simulink model "Final_project_TEMPLATE"  (R2015b)
settings: Solver=FixedStepDiscrete  StartTime=0.0  StopTime=10.0  RelTol=1e-3
InitFcn:
  | parameters
values from neighbouring files (symbols this model uses):
  Ak = 100    [parameters.m]
  b = 100    [parameters.m]
  dc_sathigh = .76    (= 0.76)    [parameters.m]
  dc_satlow = .24    (= 0.24)    [parameters.m]
  dT = 0.01    [parameters.m]
  H = 20    [parameters.m]
  L1 = 1.6    [parameters.m]
  L2 = 0.8    [parameters.m]
  m = 2000    [parameters.m]
  n_desired = 0    [parameters.m]
  pot_gain = 1    [parameters.m]
  pot_offset = 512    [parameters.m]
  R = 1/5    (= 0.2)    [parameters.m]
  S_Kd1 = .045    (= 0.045)    [parameters.m]
  S_Kd2 = 80    [parameters.m]
  S_Ki2 = 0.0001    [parameters.m]
  S_Kp1 = 0.45    [parameters.m]
  S_Kp2 = 600    [parameters.m]
  t2d = 2*pi/4000    (= 0.00157079632679)    [parameters.m]
  V_Ki = 50    [parameters.m]
  V_Kp = 5000    [parameters.m]
undefined symbols (not defined in the file or in its folder): A10, A13, A14, AN0, AN12, B, B13, B4, B6, C6, D, D11, D4, DiscIntNeverNeededParam, F15, F3, F4, G4, H4, L3, M14, N15, PA10, PA11, PA12, PA13, PA14, PA5, PA6, PA7, PA8, PA9, PB10, PB7, PC11, PC12, PC13, PC6, PD11, R10, R16, R5, R8
libraries: Conv_Lib x54, rappid_564xl_ec_toolbox x37, Veh_Sim x9, simulink x2, U_of_M_5643_blockset x1
(part 1 of 2)
settings Model: Creator=cculkin  LastModifiedBy=yiyupan
settings DataIOCC: ExternalInput=off  InitialState=off  SaveOutput=off  SignalLogging=off  SaveTime=off
settings OptimizationCC: DefaultParameterBehavior=Inlined  DataBitsets=on  OptimizeModelRefInitCode=on  LifeSpan=1
settings DebuggingCC: InheritedTsInSrcMsg=none  SingleTaskRateTransMsg=error  UnconnectedInputMsg=error  UnconnectedOutputMsg=error  UnconnectedLineMsg=error  UnknownTsInhSupMsg=error
settings HardwareCC: ProdBitPerPointer=32  ProdLargestAtomicInteger=Long  ProdLargestAtomicFloat=Double  ProdEndianess=BigEndian  ProdWordSize=32  ProdHWDeviceType=Freescale->32-bit PowerPC
settings RTWCC: SystemTargetFile=rappid564xl.tlc  MakeCommand=rappid_564xl_make_rtw  TemplateMakefile=rappid_564xl_default_tmf  PostCodeGenCommand=rappid_analyzegencode(buildInfo)  Description=RAppID Toolbox MPC564xL Code Generation Target (rappid)  GenerateReport=on  IncludeHyperlinkInReport=on  LaunchReport=on
settings CodeAppCC: IgnoreCustomStorageClasses=off
settings STFCustomTargetCC: ModelReferenceCompliant=off  ConcurrentExecutionCompliant=off  GeneratePreprocessorConditionals=Use local settings  CombineOutputUpdateFcns=on  ERTCustomFileBanners=on  SupportContinuousTime=off  SupportNonInlinedSFcns=off  MATLABClassNameForMDSCustomization=Simulink.SoftwareTarget.ERTCustomization  CPPClassGenCompliant=off  GRTInterface=off  SystemTargetFile=rappid564xl.tlc
settings ERTTargetCC: ModelReferenceCompliant=off  ParMdlRefBuildCompliant=off  CompOptLevelCompliant=off  ConcurrentExecutionCompliant=off  ERTFirstTimeCompliant=off  ModelStepFunctionPrototypeControlCompliant=off  CPPClassGenCompliant=off  UseToolchainInfoCompliant=off  InlinedParameterPlacement=NonHierarchical  ERTCustomFileTemplate=example_file_process.tlc

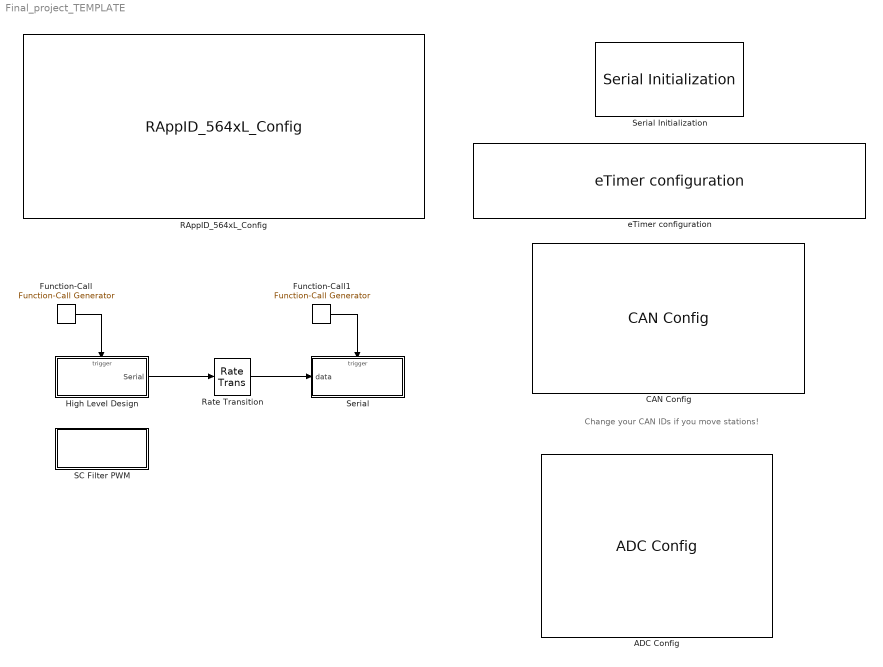
== system Final_project_TEMPLATE ==
  note: Change your CAN IDs if you move stations!
  ADC Config : rappid_564xl_ec_toolbox/MPC564xL/Motor Control Blocks/ADC Config  adc_unit=0  adc_ctu=off  adc_owr=on  adc_wls=Left  adc_clk=on  adc_ack=on  adc_ctr0_inp=off  adc_ctr0_shft=10 - Avin = 0  adc_ctr0_cmp=01  adc_ctr0_samp=3  adc_ctr1_inp=off  adc_ctr1_cmp=01  adc_ctr1_samp=1  adc_ctr1_tsens=PTAT  adc_pscr_preval=V0  adc_pscr_preconv=off
  CAN Config : rappid_564xl_ec_toolbox/MPC564xL/Communication Blocks/CAN Config  Priority=1  can_unit=A  can_unit_v2=0  can_idam=A - One full ID (standard or extended) per filter element.  can_srx_dis=1 - Self reception disabled  can_presdiv=4  can_rjw=3  can_pseg1=5  can_pseg2=5  can_clk_src=0 - The CAN engine clock source is the oscillator clock  can_lpb=0 - Loop Back disabled  can_smp=0 - One sample is used to determine the bit value  can_boff_rec=0 - Automatic recovering from Bus Off state enabled  can_tsyn=0 - Timer Sync feature disabled  can_lbuf=0 - Buffer with highest priority is transmitted first  can_lom=0 - Listen Only Mode is deactivated  can_propseg=2
  Function-Call : simulink/Ports & Subsystems/Function-Call Generator  sample_time=dT  numberOfIterations=1
  Function-Call1 : simulink/Ports & Subsystems/Function-Call Generator  sample_time=0.05  numberOfIterations=1
  High Level Design : Subsystem  TreatAsAtomicUnit=on
  RAppID_564xL_Config : rappid_564xl_ec_toolbox/MPC564xL/RAppID_564xL_Config  SystemClock=120  XTAL=40  MC_clock_60=12  MC_clock_80=16  MC_clock_120=10  SWG_clock_60=20  SWG_clock_80=13.334  SWG_clock_120=20  Compiler=CodeWarrior  MemTarget=FLASH  Part=MPC5643L  Package=144 LQFP  global_int_priority=10  base_tick_priority=11  sys_task_supress=off  exception_handlers=off  stored_mdl_name=adc_pit_block_new  freemaster_interface=Oops  freemaster_rx_pin="LINFlex_0 Rx Pin 116 : \"PB[3]\""  freemaster_tx_pin="LINFlex_0 Tx Pin 114 : \"PB[2]\""  freemaster_interface_1=Serial 0  freemaster_enable=on  freemaster_rate=115200  freemaster_tx0_pin=18 : B[2] : 114 : A14  freemaster_rx0_pin=19 : B[3] : 116 : B13  freemaster_tx1_pin=57 : D[9] : 26 : L3  freemaster_rx1_pin=29 : B[13] : 60 : R10  freemaster_can_channel=1CH  freemater_can_speed=500K  freemaster_can_msgig=0x7AA  ccp_interface=None  ccp_enable=off  ccp_can_channel=CH1 (MB 0 - 1)  ccp_can_speed=500K  ccp_can_cro_id=256  ccp_can_dto_id=257  ccp_dev_id=RappID  ccp_dev_addr=0  ccp_odt=3  ccp_daq=3  pil_enable=off  pil_bam=off  comport=4  pil_rate=115200  bam_password_def=on  bam_password=0xFEEDFACECAFEBEEF  bam_sa_cs=off  bam_start_address=0x0  bam_code_size=0x7000  cons_dspi=on  cons_can=on  cons_adc=on  cons_pwm=on  cons_ctu=on  cons_swg=on  cons_eTimer=on  cons_fm=on
  Rate Transition : RateTransition
  SC Filter PWM : Subsystem
  Serial : Subsystem  TreatAsAtomicUnit=on
  Serial Initialization : U_of_M_5643_blockset/Serial/Serial Initialization
  eTimer configuration : rappid_564xl_ec_toolbox/MPC564xL/Motor Control Blocks/eTimer configuration  SubModule=0  TimerChan=0  subMod=0  channel=0  CountMode=100 - Quadrature count mode using primary and secondary sources  CNTMODE=4  CountOnce=0 - Count repeatedly  ONCE=0  CountLength=0 - Continue counting to roll over  LENGTH=0  CountDirection=0 - Count up  DIR=0  OutputEnable=0 - The external pin is configured as an input  OEN=0  CoChanInit=00 - Other channels cannot force re-initialization of this channel  COINIT=0  StopAction=0 - Output enable is unaffected by stop mode  STPEN=0  ReloadOnCapt=00 - Do not reload the counter on a capture event  ROC=0  PrimarySource=00000 - Counter #0 input pin  PRISRC=0  PrimSrcPol=0 - True polarity  PIPS=0  SecondarySource=00001 - Counter #1 input pin  SECSRC=1  SecSrcPol=0 - True polarity  SIPS=0  FILT_CNT=0  FILT_PER=0  FILT=0  OutputMode=0000 - Software controlled  OUTMODE=0  OutputPol=0 - True polarity  OPS=0  MasterMode=0 - Disable broadcast of this channel output  MSTR=0  ForcedOutVal=0  VAL=0  CoForce=0 - Other channels cannot force this channel output  COFRC=0  CompLoad1=000 - COMP1 is never preload  CLC1=0  CompLoad2=000 - COMP2 is never preload  CLC2=0  CompareMode="00 - COMP1 and COMP2  are used when the counter is counting up"  CMPMODE=0  CaptMode1=00 - Capture disabled  CPT1MODE=0  CaptMode2=00 - Capture disabled  CPT2MODE=0  OneShCaptMode=0 - Free running mode is selected  ONESHOT=0  CaptFIFO=0  CFWM=0  CNTRinit=0  COMP1init=0  COMP2init=0  mod0ch0pin="0   : PA0  : [ 73 ] : [ T14 ]  input/output"  mod0ch1pin="1   : PA1  : [ 74 ] : [ R14 ]  input/output"  mod0ch2pin=None  mod0ch3pin=None  mod0ch4pin=None  mod0ch5pin=None  mod1ch0pin=None  mod1ch1pin=None  mod1ch2pin=None  mod1ch3pin=None  mod1ch4pin=None  mod1ch5pin=None  mod2ch0pin=None  mod2ch1pin=None  mod2ch2pin=None  mod2ch3pin=None  mod2ch4pin=None  mod2ch5pin=None  pcrNum0=0  pcrNum1=1  pcrNum2=255  pcrNum3=255  pcrNum4=255  pcrNum5=255  TCFIE=off  TCF1IE=off  TCF2IE=off  TOFIE=off  IELFIE=off  IEHFIE=off  ICF1IE=off  ICF2IE=off  INTDMA=0
  wires:
  Function-Call/1 -> High Level Design/Trigger
  Function-Call1/1 -> Serial/Trigger
  High Level Design/1(Serial) -> Rate Transition/1
  Rate Transition/1 -> Serial/1(data)

== system Final_project_TEMPLATE/High Level Design ==
  function : TriggerPort  TriggerType=function-call
  ACC : Subsystem
  Automatic Steering : Subsystem
  Constant : Constant  Value=n_desired
  Data Type Conversion : DataTypeConversion  OutDataTypeStr=single
  Inputs : Subsystem
  Outputs : Subsystem
  Vehicle : Subsystem
  Serial : Outport
  wires:
  Outputs/1("x, y, psi (Cars 1-6)") -> Serial/1
  Inputs/6(Automatic Steering Enable (GPDI 14)) -> Automatic Steering/1(Enable)
  Inputs/1("s, n, psi, us (Cars 1-6)") -> Outputs/1("s, n, psi, us (Cars 1-6)"), ACC/1(car1_6_data)
  Inputs/2(ACC_enable (GPDI 13)) -> ACC/2(ACC_enable)
  Constant/1 -> Data Type Conversion/1
  Inputs/5(Throttle (Fd)) -> ACC/4(Fd_in)
  ACC/1(Fd) -> Vehicle/1(Fd1)
  Vehicle/3(Torque_sa) -> Outputs/4(Self-Aligning Torque)
  Vehicle/1(My_car) -> ACC/3(my_car), Outputs/2("s, n, psi, us (My Car)")
  Vehicle/2(u) -> ACC/6(speed_in), Outputs/3(u (My car))
  Vehicle/4("n ") -> Automatic Steering/3(n)
  Inputs/3(Cruise Control Speed) -> ACC/5(speed_set)
  Data Type Conversion/1 -> Automatic Steering/2(n_des)
  Inputs/4(Steering Angle (delta)) -> Automatic Steering/4(delta), Vehicle/2(delta)
  Automatic Steering/1(Auto_torque) -> Outputs/5(Auto Torque)

== system Final_project_TEMPLATE/SC Filter PWM ==
  Constant1 : Constant  Value=1e6  OutDataTypeStr=uint32
  Constant2 : Constant  Value=0  OutDataTypeStr=uint32
  Constant3 : Constant  Value=50  OutDataTypeStr=uint32
  Simple PWM Output : rappid_564xl_ec_toolbox/MPC564xL/Motor Control Blocks/Simple PWM Output  Priority=1  pwmModule=0  pwmMod=0  SubModule=1  subMod=1  InitFreq=1000000  resolution=1 %  resValue=1  InitDutyA=0  InitDutyB=50  align=A B - edge aligned  PhaseShift_A=0  PhaseShift=0  Phase_A=0  Phase_B=0  centered=0  DoubleS=off  doubleSw=off  debugSw=off  debug_mode=0  pin_A0=None  pin_B0=None  pin_X0=None  pin_A1=None  pin_B1="38  : PC6  : [ 142 ] : [ D4 ]"  pin_X1=None  pin_A2=None  pin_B2=None  pin_X2=None  pin_A3=None  pin_B3=None  pin_X3=None  pin1_A0=None  pin1_B0=None  pin1_X0=None  pin1_A1=None  pin1_B1=None  pin1_X1=None  pin1_A2=None  pin1_B2=None  pin1_X2=None  pin1_A3=None  pin1_B3=None  pin1_X3=None  pcrNumA=255  pcrNumB=38  pcrNumX=255  polA=off  polB=off  polX=off  octrl=0  syncFrom0=off  masterSync=0  outVal0=off  outVal1=off  outVal2=off  outVal3=off  outVal4=on  outVal5=on  outTrig=48
  wires:
  Constant1/1 -> Simple PWM Output/1
  Constant2/1 -> Simple PWM Output/2
  Constant3/1 -> Simple PWM Output/3

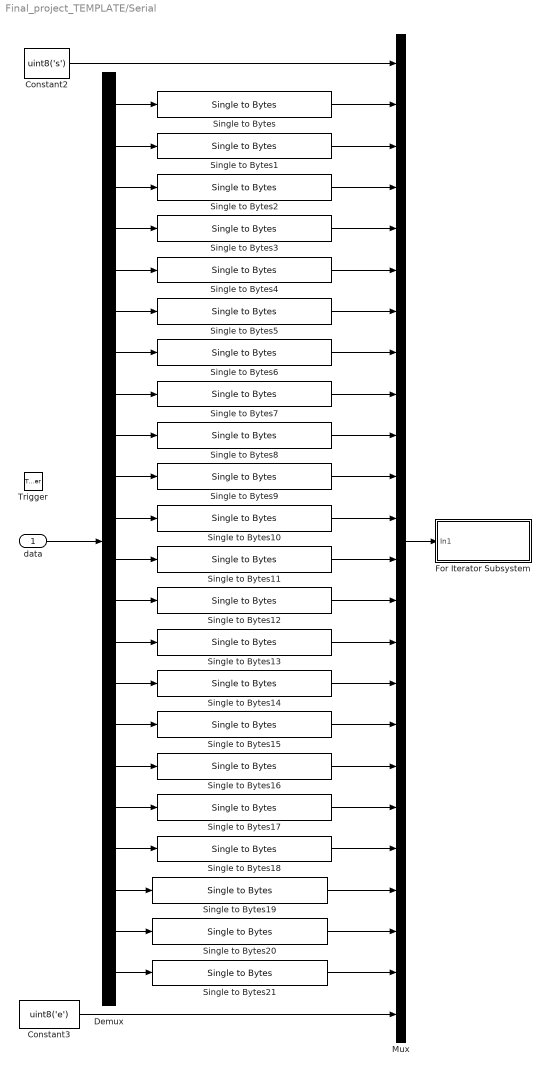
== system Final_project_TEMPLATE/Serial ==
  data : Inport
  Trigger : TriggerPort  TriggerType=function-call
  Constant2 : Constant  Value=uint8('s')  OutDataTypeStr=uint8
  Constant3 : Constant  Value=uint8('e')  OutDataTypeStr=uint8
  Demux : Demux  Outputs=22
  For Iterator Subsystem : Subsystem
  Mux : Mux  Inputs=24
  Single to Bytes{,1..21} (22 alike) : Conv_Lib/Single to Bytes
  wires:
  Constant2/1 -> Mux/1
  Single to Bytes/1 -> Mux/2
  Single to Bytes1/1 -> Mux/3
  Single to Bytes2/1 -> Mux/4
  Single to Bytes3/1 -> Mux/5
  Single to Bytes4/1 -> Mux/6
  Single to Bytes5/1 -> Mux/7
  Single to Bytes6/1 -> Mux/8
  Single to Bytes7/1 -> Mux/9
  Single to Bytes8/1 -> Mux/10
  Single to Bytes9/1 -> Mux/11
  Single to Bytes10/1 -> Mux/12
  Single to Bytes11/1 -> Mux/13
  Single to Bytes12/1 -> Mux/14
  Single to Bytes13/1 -> Mux/15
  Single to Bytes15/1 -> Mux/17
  Single to Bytes16/1 -> Mux/18
  Single to Bytes17/1 -> Mux/19
  Mux/1 -> For Iterator Subsystem/1(In1)
  Demux/1 -> Single to Bytes/1
  Demux/2 -> Single to Bytes1/1
  Demux/3 -> Single to Bytes2/1
  Demux/4 -> Single to Bytes3/1
  Demux/5 -> Single to Bytes4/1
  Demux/6 -> Single to Bytes5/1
  Demux/7 -> Single to Bytes6/1
  Demux/8 -> Single to Bytes7/1
  Demux/9 -> Single to Bytes8/1
  Demux/10 -> Single to Bytes9/1
  Demux/11 -> Single to Bytes10/1
  Demux/12 -> Single to Bytes11/1
  Demux/13 -> Single to Bytes12/1
  Demux/14 -> Single to Bytes13/1
  Demux/15 -> Single to Bytes14/1
  Demux/16 -> Single to Bytes15/1
  Demux/17 -> Single to Bytes16/1
  Demux/18 -> Single to Bytes17/1
  data/1 -> Demux/1
  Single to Bytes14/1 -> Mux/16
  Demux/19 -> Single to Bytes18/1
  Demux/20 -> Single to Bytes19/1
  Demux/21 -> Single to Bytes20/1
  Demux/22 -> Single to Bytes21/1
  Single to Bytes18/1 -> Mux/20
  Single to Bytes19/1 -> Mux/21
  Single to Bytes20/1 -> Mux/22
  Single to Bytes21/1 -> Mux/23
  Constant3/1 -> Mux/24

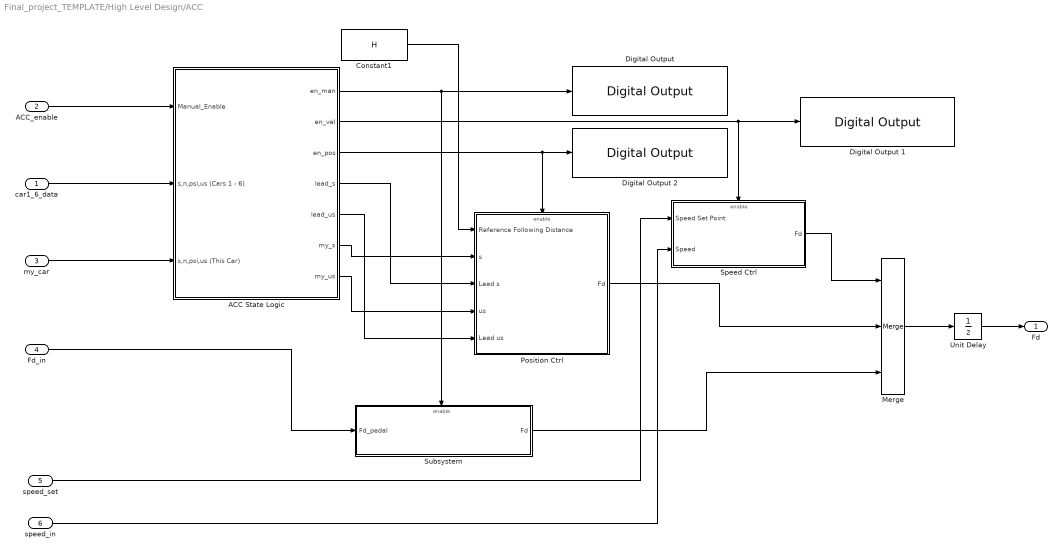
== system Final_project_TEMPLATE/High Level Design/ACC ==
  car1_6_data : Inport
  ACC_enable : Inport  Port=2
  my_car : Inport  Port=3
  Fd_in : Inport  Port=4
  speed_set : Inport  Port=5
  speed_in : Inport  Port=6
  ACC State Logic : Subsystem
  Constant1 : Constant  Value=H
  "Digital Output " : rappid_564xl_ec_toolbox/MPC564xL/General Purpose Blocks/Digital Output   gpio_outputs="43  : PC11 : [ 80 ] : [ M14 ]"  pinNum=[ 80 ]  pcrNum=43
  Digital Output 1 : rappid_564xl_ec_toolbox/MPC564xL/General Purpose Blocks/Digital Output   gpio_outputs="44  : PC12 : [ 82 ] : [ N15 ]"  pinNum=[ 82 ]  pcrNum=44
  Digital Output 2 : rappid_564xl_ec_toolbox/MPC564xL/General Purpose Blocks/Digital Output   gpio_outputs="45  : PC13 : [ 101 ] : [ F15 ]"  pinNum=[ 101 ]  pcrNum=45
  Merge : Merge  Inputs=3
  Position Ctrl : Subsystem  TreatAsAtomicUnit=on
  Speed Ctrl : Subsystem  TreatAsAtomicUnit=on
  Subsystem : Subsystem
  Unit Delay : UnitDelay  SampleTime=-1
  Fd : Outport
  wires:
  my_car/1 -> ACC State Logic/3(s,n,psi,us (This Car))
  car1_6_data/1 -> ACC State Logic/2(s,n,psi,us (Cars 1 - 6))
  ACC_enable/1 -> ACC State Logic/1(Manual_Enable)
  ACC State Logic/3(en_pos) -> Digital Output 2/1, Position Ctrl/Enable
  ACC State Logic/2(en_vel) -> Speed Ctrl/Enable, Digital Output 1/1
  Speed Ctrl/1(Fd) -> Merge/1
  Position Ctrl/1(Fd) -> Merge/2
  Merge/1 -> Unit Delay/1
  Fd_in/1 -> Subsystem/1(Fd_pedal)
  ACC State Logic/1(en_man) -> "Digital Output "/1, Subsystem/Enable
  Subsystem/1(Fd) -> Merge/3
  ACC State Logic/4(lead_s) -> Position Ctrl/3(Lead s)
  ACC State Logic/5(lead_us) -> Position Ctrl/5(Lead us)
  ACC State Logic/6(my_s) -> Position Ctrl/2(s)
  ACC State Logic/7(my_us) -> Position Ctrl/4(us)
  Constant1/1 -> Position Ctrl/1(Reference Following Distance)
  speed_set/1 -> Speed Ctrl/1(Speed Set Point)
  speed_in/1 -> Speed Ctrl/2(Speed)
  Unit Delay/1 -> Fd/1

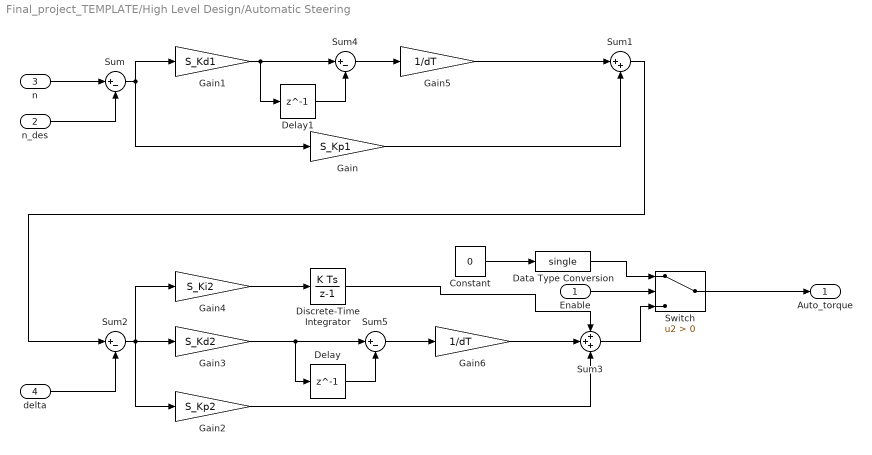
== system Final_project_TEMPLATE/High Level Design/Automatic Steering ==
  Enable : Inport
  n_des : Inport  Port=2
  n : Inport  Port=3
  delta : Inport  Port=4
  Constant : Constant  Value=0
  Data Type Conversion : DataTypeConversion  OutDataTypeStr=single
  Delay : Delay  DelayLength=1
  Delay1 : Delay  DelayLength=1
  Discrete-Time Integrator : DiscreteIntegrator  SampleTime=-1  ICPrevOutput=DiscIntNeverNeededParam  ICPrevScaledInput=DiscIntNeverNeededParam
  Gain : Gain  Gain=S_Kp1
  Gain1 : Gain  Gain=S_Kd1
  Gain2 : Gain  Gain=S_Kp2
  Gain3 : Gain  Gain=S_Kd2
  Gain4 : Gain  Gain=S_Ki2
  Gain5 : Gain  Gain=1/dT
  Gain6 : Gain  Gain=1/dT
  Sum{,2,4..5} (4 alike) : Sum  Inputs=|+-
  Sum1 : Sum  Inputs=|++
  Sum3 : Sum  Inputs=+++
  Switch : Switch  Criteria=u2 > Threshold
  Auto_torque : Outport
  wires:
  n/1 -> Sum/1
  n_des/1 -> Sum/2
  Gain1/1 -> Delay1/1, Sum4/1
  Sum/1 -> Gain/1, Gain1/1
  Sum4/1 -> Gain5/1
  Gain/1 -> Sum1/2
  Sum2/1 -> Gain4/1, Gain2/1, Gain3/1
  Sum3/1 -> Switch/3
  Enable/1 -> Switch/2
  Constant/1 -> Data Type Conversion/1
  Gain4/1 -> Discrete-Time Integrator/1
  Discrete-Time Integrator/1 -> Sum3/1
  Gain6/1 -> Sum3/2
  Gain2/1 -> Sum3/3
  Data Type Conversion/1 -> Switch/1
  Switch/1 -> Auto_torque/1
  Sum1/1 -> Sum2/1
  delta/1 -> Sum2/2
  Delay1/1 -> Sum4/2
  Gain5/1 -> Sum1/1
  Gain3/1 -> Delay/1, Sum5/1
  Sum5/1 -> Gain6/1
  Delay/1 -> Sum5/2

== system Final_project_TEMPLATE/High Level Design/Inputs ==
  Data Type Conversion : DataTypeConversion  OutDataTypeStr=single
  Digital Input : rappid_564xl_ec_toolbox/MPC564xL/General Purpose Blocks/Digital Input  gpio_outputs="13  : PA13 : [ 136 ] : [ C6 ]"  pinNum=[ 136 ]  pcrNum=13
  Digital Input1 : rappid_564xl_ec_toolbox/MPC564xL/General Purpose Blocks/Digital Input  gpio_outputs="14  : PA14 : [ 143 ] : [ B4 ]"  pinNum=[ 143 ]  pcrNum=14
  Gain : Gain  Gain=-1
  Other Cars : Subsystem
  Scale : Gain  Gain=R
  Select Speed (GPDI 5-12) : Subsystem
  Steering angle (QD) : Subsystem
  Throttle (ADC) : Subsystem
  "s, n, psi, us (Cars 1-6)" : Outport
  ACC_enable (GPDI 13) : Outport  Port=2
  Cruise Control Speed : Outport  Port=3
  Steering Angle (delta) : Outport  Port=4
  Throttle (Fd) : Outport  Port=5
  Automatic Steering Enable (GPDI 14) : Outport  Port=6
  wires:
  Other Cars/1("s, n, psi, us (Cars 1-6)1") -> "s, n, psi, us (Cars 1-6)"/1
  Select Speed (GPDI 5-12)/1(Speed) -> Scale/1
  Throttle (ADC)/1(Fd) -> Throttle (Fd)/1
  Steering angle (QD)/1(delta (deg)) -> Gain/1
  Scale/1 -> Data Type Conversion/1
  Digital Input/1 -> ACC_enable (GPDI 13)/1
  Digital Input1/1 -> Automatic Steering Enable (GPDI 14)/1
  Data Type Conversion/1 -> Cruise Control Speed/1
  Gain/1 -> Steering Angle (delta)/1

== system Final_project_TEMPLATE/High Level Design/Outputs ==
  "s, n, psi, us (Cars 1-6)" : Inport
  "s, n, psi, us (My Car)" : Inport  Port=2
  u (My car) : Inport  Port=3
  Self-Aligning Torque : Inport  Port=4
  Auto Torque : Inport  Port=5
  Extract x,y,psi : Subsystem
  Extract x,y,psi (Cars 1 - 6) : Subsystem
  Mux : Mux  Inputs=3
  Output Torque : Subsystem
  Sum1 : Sum  Inputs=|--
  Tx CAN : Subsystem
  "x, y, psi (Cars 1-6)" : Outport
  wires:
  Self-Aligning Torque/1 -> Sum1/1
  Auto Torque/1 -> Sum1/2
  Sum1/1 -> Output Torque/1(Torque)
  "s, n, psi, us (Cars 1-6)"/1 -> Extract x,y,psi (Cars 1 - 6)/1(s,n,psi,us (Cars 1 - 6))
  Extract x,y,psi/1(x,y,psi) -> Mux/1
  Mux/1 -> "x, y, psi (Cars 1-6)"/1
  u (My car)/1 -> Mux/2
  Extract x,y,psi (Cars 1 - 6)/1(x,y,psi (Cars 1 - 6)) -> Mux/3
  "s, n, psi, us (My Car)"/1 -> Tx CAN/1(s,n,psi,us), Extract x,y,psi/1(s,n,psi,us)

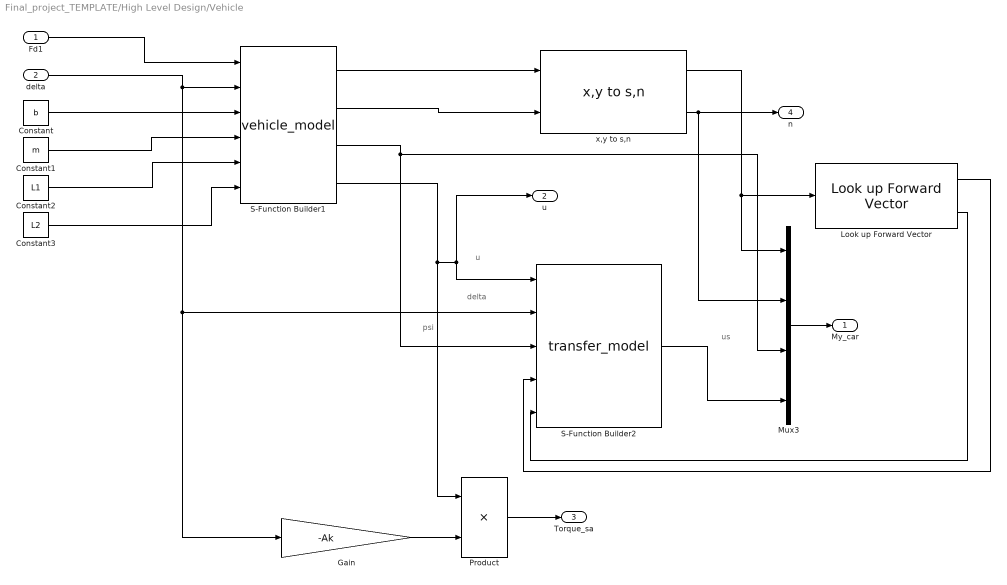
== system Final_project_TEMPLATE/High Level Design/Vehicle ==
  note: us
  note: psi
  note: delta
  note: u
  Fd1 : Inport
  delta : Inport  Port=2
  Constant : Constant  Value=b  OutDataTypeStr=single
  Constant1 : Constant  Value=m  OutDataTypeStr=single
  Constant2 : Constant  Value=L1  OutDataTypeStr=single
  Constant3 : Constant  Value=L2  OutDataTypeStr=single
  Gain : Gain  Gain=-Ak
  Look up Forward Vector : Veh_Sim/Look up Forward Vector  SystemSampleTime=-1
  Mux3 : Mux
  Product : Product
  S-Function Builder1 : S-Function  InitFcn=try, set_param(gcb,'FunctionName','vehicle_model'), end  FunctionName=vehicle_model  SFunctionModules=vehicle_model_wrapper  SFunctionDeploymentMode=off  EnableBusSupport=off  mask(S-Function Builder){}
      mask help: Simulink:masks:SFunctionBuilder_MD
      mask init:
      | val = [[.9  0.75 0.75 1 1 .9 .9 1]',[1 1 0.75 0.75 .9 .9 1 .9]'];try , sys = get_param(gcb,'SfunBuilderFcnName');if isempty(sys), sys = get_param(gcb,'FunctionName'); end,catch, sys = get_param(gcb,'FunctionName'); end
      settings: CopyFcn=set_param(gcbh,'LinkStatus','none')  PreSaveFcn=try, set_param(gcb,'FunctionName','vehicle_model'), end  OpenFcn=sfunctionwizard(gcbh)
      mask Display: plot(val(:,1),val(:,2)),disp(sys), port_label('input',1,'u0'), port_label('input',2,'u1'), port_label('input',3,'u2'), port_label('input',4,'u3'), port_label('input',5,'u4'), port_label('input',6,'u5'), port_label('output',1,'x'), port_label('output',2,'y'), port_label('output',3,'psi'), port_label('output',4,'u')
  S-Function Builder2 : S-Function  InitFcn=try, set_param(gcb,'FunctionName','transfer_model'), end  FunctionName=transfer_model  SFunctionModules=transfer_model_wrapper  SFunctionDeploymentMode=off  EnableBusSupport=off  mask(S-Function Builder){}
      mask help: Simulink:masks:SFunctionBuilder_MD
      mask init: same as Final_project_TEMPLATE/High Level Design/Vehicle/S-Function Builder1
      settings: CopyFcn=set_param(gcbh,'LinkStatus','none')  PreSaveFcn=try, set_param(gcb,'FunctionName','transfer_model'), end  OpenFcn=sfunctionwizard(gcbh)
      mask Display: plot(val(:,1),val(:,2)),disp(sys), port_label('input',1,'u0'), port_label('input',2,'u1'), port_label('input',3,'u2'), port_label('input',4,'u3'), port_label('input',5,'u4'), port_label('output',1,'y0')
  x,y to s,n : Veh_Sim/x,y to s,n  SystemSampleTime=-1
  My_car : Outport
  u : Outport  Port=2
  Torque_sa : Outport  Port=3
  "n " : Outport  Port=4
  wires:
  S-Function Builder1/1 -> x,y to s,n/1
  S-Function Builder1/2 -> x,y to s,n/2
  S-Function Builder1/3 -> S-Function Builder2/3, Mux3/3
  delta/1 -> S-Function Builder1/2, Gain/1, S-Function Builder2/2
  Constant/1 -> S-Function Builder1/3
  Constant1/1 -> S-Function Builder1/4
  Constant3/1 -> S-Function Builder1/6
  Fd1/1 -> S-Function Builder1/1
  x,y to s,n/1 -> Look up Forward Vector/1, Mux3/1
  Look up Forward Vector/1 -> S-Function Builder2/4
  Look up Forward Vector/2 -> S-Function Builder2/5
  S-Function Builder1/4 -> Product/1, S-Function Builder2/1, u/1
  x,y to s,n/2 -> "n "/1, Mux3/2
  Gain/1 -> Product/2
  Product/1 -> Torque_sa/1
  Mux3/1 -> My_car/1
  S-Function Builder2/1 -> Mux3/4
  Constant2/1 -> S-Function Builder1/5

== system Final_project_TEMPLATE/Serial/For Iterator Subsystem ==
  In1 : Inport
  Data Type Conversion : DataTypeConversion  OutDataTypeStr=uint8
  For Iterator : ForIterator  IterationLimit=90  IndexMode=Zero-based  IterationVariableDataType=int8
  Index Vector : MultiPortSwitch  DataPortOrder=Zero-based contiguous  Inputs=1  zeroidx=on
  S-Function : S-Function  FunctionName=SerialSend  SFunctionDeploymentMode=off  EnableBusSupport=off
      mask Display:
      | patch([0 0 1 1], [0 1 1 0], [255/255 255/255 0])
      | patch([0 0 0.05 0.05], [0 1 1 0], [0 0 255/255])
      | patch([1 1 0.95 0.95], [0 1 1 0], [0 0 255/255])
      | 
      | text (0.52, 0.8, ['Serial Send'], 'horizontalAlignment', 'center');
      | %text (0.5, .5, ['System Clock MHz: ' get_param(gcb,'SystemClock')], 'horizontalAlignment', 'center');
      | %text (0.5, .35, ['Baud Rate: ' get_param(gcb,'BaudRate')], 'horizontalAlignment', 'center');
      | text(0.5, 0.1, 'The University of Michigan', 'horizontalAlignment', 'center');
  wires:
  In1/1 -> Index Vector/2
  Index Vector/1 -> Data Type Conversion/1
  For Iterator/1 -> Index Vector/1
  Data Type Conversion/1 -> S-Function/1

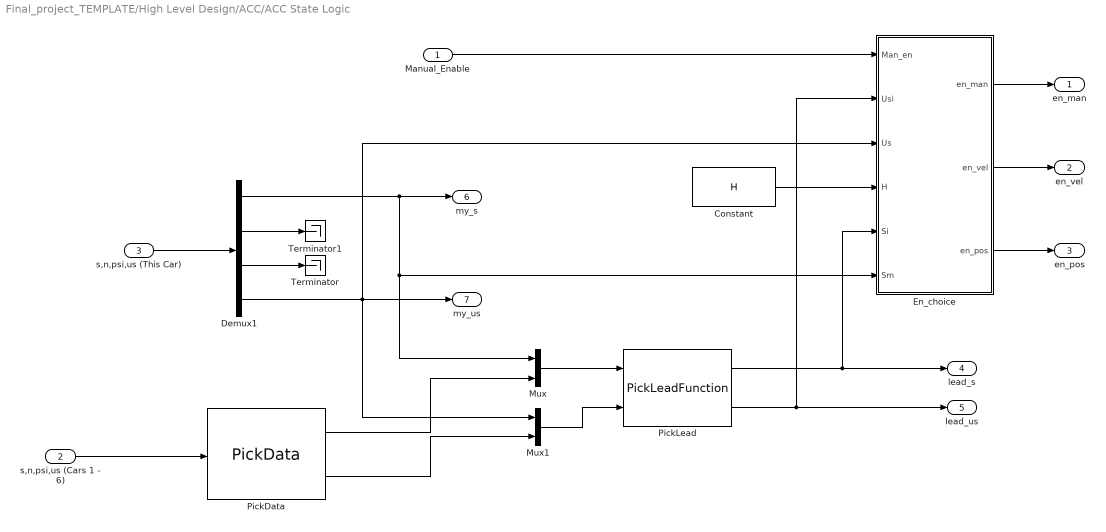
== system Final_project_TEMPLATE/High Level Design/ACC/ACC State Logic ==
  Manual_Enable : Inport
  s,n,psi,us (Cars 1 - 6) : Inport  Port=2
  s,n,psi,us (This Car) : Inport  Port=3
  Constant : Constant  Value=H
  Demux1 : Demux
  En_choice : Stateflow chart  TreatAsAtomicUnit=on
  Mux : Mux  Inputs=2
  Mux1 : Mux  Inputs=2
  PickData : S-Function  InitFcn=try, set_param(gcb,'FunctionName','PickData'), end  FunctionName=PickData  SFunctionModules=PickData_wrapper  SFunctionDeploymentMode=off  EnableBusSupport=off  mask(S-Function Builder){}
      mask help: Simulink:masks:SFunctionBuilder_MD
      mask init: same as Final_project_TEMPLATE/High Level Design/Vehicle/S-Function Builder1
      settings: CopyFcn=set_param(gcbh,'LinkStatus','none')  PreSaveFcn=try, set_param(gcb,'FunctionName','PickData'), end  OpenFcn=sfunctionwizard(gcbh)
      mask Display:
      | plot(val(:,1),val(:,2))
      | disp(sys)
      | port_label('input',1,'CarsIn')
      | port_label('output',1,'CarS')
      | port_label('output',2,'CarUS')
  PickLead : S-Function  InitFcn=try, set_param(gcb,'FunctionName','PickLeadFunction'), end  FunctionName=PickLeadFunction  SFunctionModules=PickLeadFunction_wrapper  SFunctionDeploymentMode=off  EnableBusSupport=off  mask(S-Function Builder){}
      mask help: Simulink:masks:SFunctionBuilder_MD
      mask init: same as Final_project_TEMPLATE/High Level Design/Vehicle/S-Function Builder1
      settings: CopyFcn=set_param(gcbh,'LinkStatus','none')  PreSaveFcn=try, set_param(gcb,'FunctionName','PickLeadFunction'), end  OpenFcn=sfunctionwizard(gcbh)
      mask Display: plot(val(:,1),val(:,2)),disp(sys), port_label('input',1,'Scar'), port_label('input',2,'UScar'), port_label('output',1,'Ls'), port_label('output',2,'Lus')
  Terminator : Terminator
  Terminator1 : Terminator
  en_man : Outport
  en_vel : Outport  Port=2
  en_pos : Outport  Port=3
  lead_s : Outport  Port=4
  lead_us : Outport  Port=5
  my_s : Outport  Port=6
  my_us : Outport  Port=7
  wires:
  s,n,psi,us (This Car)/1 -> Demux1/1
  s,n,psi,us (Cars 1 - 6)/1 -> PickData/1
  Mux/1 -> PickLead/1
  PickData/1 -> Mux/2
  Demux1/4 -> my_us/1, En_choice/3(Us), Mux1/1
  Mux1/1 -> PickLead/2
  PickData/2 -> Mux1/2
  PickLead/1 -> En_choice/5(Si), lead_s/1
  PickLead/2 -> En_choice/2(Usi), lead_us/1
  Manual_Enable/1 -> En_choice/1(Man_en)
  En_choice/2(en_vel) -> en_vel/1
  En_choice/3(en_pos) -> en_pos/1
  En_choice/1(en_man) -> en_man/1
  Demux1/1 -> my_s/1, En_choice/6(Sm), Mux/1
  Demux1/3 -> Terminator/1
  Demux1/2 -> Terminator1/1
  Constant/1 -> En_choice/4(H)

== system Final_project_TEMPLATE/High Level Design/ACC/Position Ctrl ==
  note: u
  Reference Following Distance : Inport
  s : Inport  Port=2
  Lead s : Inport  Port=3
  us : Inport  Port=4
  Lead us : Inport  Port=5
  Enable : EnablePort
  D-gain : Gain  Gain=2.45*m  SaturateOnIntegerOverflow=on  OutDataTypeStr=Inherit: Same as input  ParamDataTypeStr=Inherit: Same as input
  Feed-forward : Gain  Gain=b  SaturateOnIntegerOverflow=on  OutDataTypeStr=Inherit: Same as input  ParamDataTypeStr=Inherit: Same as input
  P-gain : Gain  Gain=-1.5*m  SaturateOnIntegerOverflow=on  OutDataTypeStr=Inherit: Same as input  ParamDataTypeStr=Inherit: Same as input
  Sum1 : Sum  Inputs=|++  SaturateOnIntegerOverflow=on
  Sum2 : Sum  Inputs=+-|  SaturateOnIntegerOverflow=on
  Sum3 : Sum  Inputs=|+-  SaturateOnIntegerOverflow=on
  Sum4 : Sum  Inputs=|+-  SaturateOnIntegerOverflow=on
  Sum5 : Sum  Inputs=|++  OutDataTypeStr=single  SaturateOnIntegerOverflow=on
  Fd : Outport
  wires:
  Sum1/1 -> Sum5/1
  Sum5/1 -> Fd/1  "F"
  Feed-forward/1 -> Sum5/2
  Sum4/1 -> D-gain/1
  Lead us/1 -> Feed-forward/1, Sum4/1
  us/1 -> Sum4/2
  D-gain/1 -> Sum1/2
  P-gain/1 -> Sum1/1
  Sum2/1 -> P-gain/1
  Sum3/1 -> Sum2/2  "head-way"
  Reference Following Distance/1 -> Sum2/1  "desired distance"
  s/1 -> Sum3/2
  Lead s/1 -> Sum3/1

== system Final_project_TEMPLATE/High Level Design/ACC/Speed Ctrl ==
  Speed Set Point : Inport
  Speed : Inport  Port=2
  Enable : EnablePort
  Gain : Gain  Gain=b  SaturateOnIntegerOverflow=on  OutDataTypeStr=Inherit: Same as input  ParamDataTypeStr=Inherit: Same as input
  PI : Subsystem
  Sum : Sum  Inputs=++|  OutDataTypeStr=single  SaturateOnIntegerOverflow=on
  Sum1 : Sum  Inputs=|+-  SaturateOnIntegerOverflow=on
  Fd : Outport
  wires:
  PI/1(U) -> Sum/2
  Gain/1 -> Sum/1
  Sum1/1 -> PI/1(Error)
  Speed/1 -> Sum1/2
  Speed Set Point/1 -> Sum1/1, Gain/1  "desired speed"
  Sum/1 -> Fd/1  "Fd"

== system Final_project_TEMPLATE/High Level Design/ACC/Subsystem ==
  Fd_pedal : Inport
  Enable : EnablePort
  Fd : Outport
  wires:
  Fd_pedal/1 -> Fd/1

== system Final_project_TEMPLATE/High Level Design/Inputs/Other Cars ==
  "1 for GSI vehicle only, 0 for ALL student vehicles 1" : Constant  Value=0
  Car 1 : Subsystem
  Car 2 : Subsystem
  Car 3 : Subsystem
  Car 4 : Subsystem
  Car 5 : Subsystem
  Car 6 : Subsystem
  GSI Car (4)1 : Subsystem
  Mux : Mux  Inputs=6
  Mux2 : Mux  Inputs=2
  Switch1 : Switch  Criteria=u2 ~= 0
  Zeros (20)1 : Subsystem
  "s, n, psi, us (Cars 1-6)1" : Outport
  wires:
  GSI Car (4)1/1(s,n,psi,us) -> Mux2/1
  Zeros (20)1/1(Zeros) -> Mux2/2
  Mux2/1 -> Switch1/1
  Switch1/1 -> "s, n, psi, us (Cars 1-6)1"/1
  Mux/1 -> Switch1/3
  "1 for GSI vehicle only, 0 for ALL student vehicles 1"/1 -> Switch1/2
  Car 1/1(s,n,psi,us) -> Mux/1
  Car 2/1(s,n,psi,us) -> Mux/2
  Car 3/1(s,n,psi,us) -> Mux/3
  Car 4/1(s,n,psi,us) -> Mux/4
  Car 5/1(s,n,psi,us) -> Mux/5
  Car 6/1(s,n,psi,us) -> Mux/6

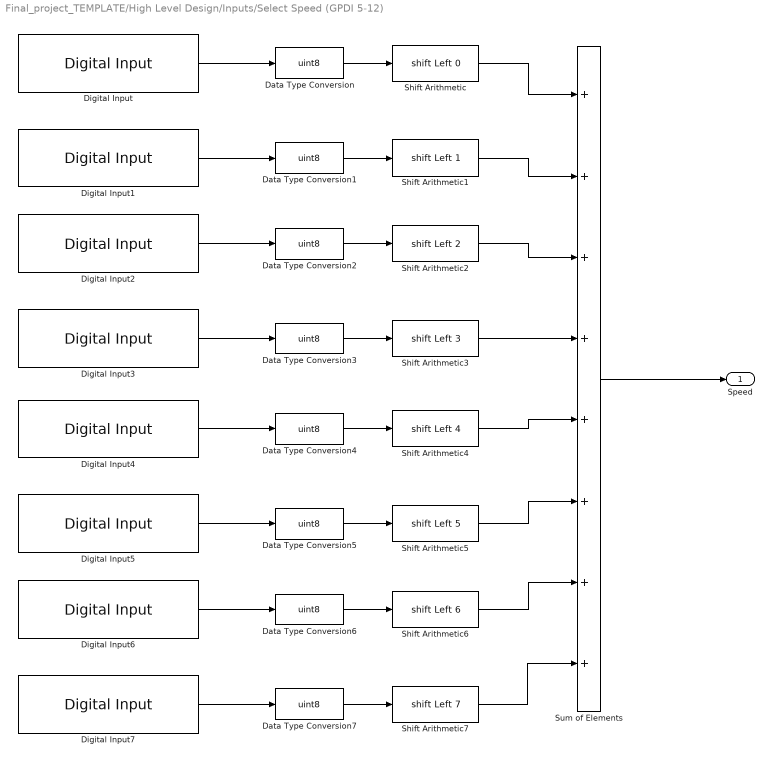
== system Final_project_TEMPLATE/High Level Design/Inputs/Select Speed (GPDI 5-12) ==
  Data Type Conversion{,1..7} (8 alike) : DataTypeConversion  OutDataTypeStr=uint8
  Digital Input : rappid_564xl_ec_toolbox/MPC564xL/General Purpose Blocks/Digital Input  gpio_outputs="5   : PA5  : [ 14 ] : [ H4 ]"  pinNum=[ 14 ]  pcrNum=5
  Digital Input1 : rappid_564xl_ec_toolbox/MPC564xL/General Purpose Blocks/Digital Input  gpio_outputs="6   : PA6  : [ 2 ] : [ G4 ]"  pinNum=[ 2 ]  pcrNum=6
  Digital Input2 : rappid_564xl_ec_toolbox/MPC564xL/General Purpose Blocks/Digital Input  gpio_outputs="7   : PA7  : [ 10 ] : [ F3 ]"  pinNum=[ 10 ]  pcrNum=7
  Digital Input3 : rappid_564xl_ec_toolbox/MPC564xL/General Purpose Blocks/Digital Input  gpio_outputs="8   : PA8  : [ 12 ] : [ F4 ]"  pinNum=[ 12 ]  pcrNum=8
  Digital Input4 : rappid_564xl_ec_toolbox/MPC564xL/General Purpose Blocks/Digital Input  gpio_outputs="9   : PA9  : [ 134 ] : [ B6 ]"  pinNum=[ 134 ]  pcrNum=9
  Digital Input5 : rappid_564xl_ec_toolbox/MPC564xL/General Purpose Blocks/Digital Input  gpio_outputs="10  : PA10  : [ 118 ] : [ A13 ]"  pinNum=[ 118 ]  pcrNum=10
  Digital Input6 : rappid_564xl_ec_toolbox/MPC564xL/General Purpose Blocks/Digital Input  gpio_outputs="11  : PA11 : [ 120 ] : [ D11 ]"  pinNum=[ 120 ]  pcrNum=11
  Digital Input7 : rappid_564xl_ec_toolbox/MPC564xL/General Purpose Blocks/Digital Input  gpio_outputs="12  : PA12 : [ 122 ] : [ A10 ]"  pinNum=[ 122 ]  pcrNum=12
  Shift Arithmetic : ArithShift  BitShiftDirection=Left
  Shift Arithmetic1 : ArithShift  BitShiftNumber=1  BitShiftDirection=Left
  Shift Arithmetic2 : ArithShift  BitShiftNumber=2  BitShiftDirection=Left
  Shift Arithmetic3 : ArithShift  BitShiftNumber=3  BitShiftDirection=Left
  Shift Arithmetic4 : ArithShift  BitShiftNumber=4  BitShiftDirection=Left
  Shift Arithmetic5 : ArithShift  BitShiftNumber=5  BitShiftDirection=Left
  Shift Arithmetic6 : ArithShift  BitShiftNumber=6  BitShiftDirection=Left
  Shift Arithmetic7 : ArithShift  BitShiftNumber=7  BitShiftDirection=Left
  Sum of Elements : Sum  Inputs=++++++++
  Speed : Outport
  wires:
  Shift Arithmetic1/1 -> Sum of Elements/2
  Digital Input1/1 -> Data Type Conversion1/1
  Shift Arithmetic2/1 -> Sum of Elements/3
  Shift Arithmetic/1 -> Sum of Elements/1
  Shift Arithmetic3/1 -> Sum of Elements/4
  Data Type Conversion3/1 -> Shift Arithmetic3/1
  Data Type Conversion2/1 -> Shift Arithmetic2/1
  Digital Input3/1 -> Data Type Conversion3/1
  Digital Input2/1 -> Data Type Conversion2/1
  Data Type Conversion/1 -> Shift Arithmetic/1
  Digital Input/1 -> Data Type Conversion/1
  Data Type Conversion1/1 -> Shift Arithmetic1/1
  Sum of Elements/1 -> Speed/1
  Shift Arithmetic5/1 -> Sum of Elements/6
  Digital Input5/1 -> Data Type Conversion5/1
  Shift Arithmetic6/1 -> Sum of Elements/7
  Shift Arithmetic4/1 -> Sum of Elements/5
  Shift Arithmetic7/1 -> Sum of Elements/8
  Data Type Conversion7/1 -> Shift Arithmetic7/1
  Data Type Conversion6/1 -> Shift Arithmetic6/1
  Digital Input7/1 -> Data Type Conversion7/1
  Digital Input6/1 -> Data Type Conversion6/1
  Data Type Conversion4/1 -> Shift Arithmetic4/1
  Digital Input4/1 -> Data Type Conversion4/1
  Data Type Conversion5/1 -> Shift Arithmetic5/1

== system Final_project_TEMPLATE/High Level Design/Inputs/Steering angle (QD) ==
  Conversion Subsystem : Subsystem
  Gain : Gain  Gain=0.04
  eTimer CNTR Register Read : rappid_564xl_ec_toolbox/MPC564xL/Motor Control Blocks/eTimer CNTR Register Read  SubModule=0  TimerChan=0  subMod=0  channel=0
  delta (deg) : Outport
  wires:
  eTimer CNTR Register Read/1 -> Conversion Subsystem/1(Encoder Counts)
  Conversion Subsystem/1(Haptic Wheel Position (degree)) -> Gain/1
  Gain/1 -> delta (deg)/1

== system Final_project_TEMPLATE/High Level Design/Inputs/Throttle (ADC) ==
  ADC Channel : rappid_564xl_ec_toolbox/MPC564xL/Motor Control Blocks/ADC Channel  adc_unit=0  adc_chan0=older  adc_chan0_v2=23 : PB7 : [43] : [R5] : AN0  adc_chan1=older  adc_chan1_v2=26 : PB10 : [53] : [R8] : AN12  simulate=off  interrupt=off  adc_mode=Normal  adc_presample=off
  Constant : Constant  Value=pot_offset  OutDataTypeStr=single
  Gain : Gain  Gain=pot_gain
  Subtract : Sum  Inputs=+-
  Fd : Outport
  wires:
  ADC Channel/1 -> Subtract/1
  Constant/1 -> Subtract/2
  Subtract/1 -> Gain/1
  Gain/1 -> Fd/1

== system Final_project_TEMPLATE/High Level Design/Outputs/Extract x,y,psi ==
  s,n,psi,us : Inport
  Demux : Demux
  Mux : Mux  Inputs=3
  Terminator : Terminator
  s,n to x,y : Veh_Sim/s,n to x,y  SystemSampleTime=-1
  x,y,psi : Outport
  wires:
  Demux/1 -> s,n to x,y/1
  Demux/2 -> s,n to x,y/2
  s,n,psi,us/1 -> Demux/1
  s,n to x,y/1 -> Mux/1
  s,n to x,y/2 -> Mux/2
  Demux/3 -> Mux/3
  Mux/1 -> x,y,psi/1
  Demux/4 -> Terminator/1

== system Final_project_TEMPLATE/High Level Design/Outputs/Extract x,y,psi (Cars 1 - 6) ==
  s,n,psi,us (Cars 1 - 6) : Inport
  Demux : Demux  Outputs=6
  Extract x,y,psi : Subsystem
  Extract x,y,psi1 : Subsystem
  Extract x,y,psi2 : Subsystem
  Extract x,y,psi3 : Subsystem
  Extract x,y,psi4 : Subsystem
  Extract x,y,psi5 : Subsystem
  Mux : Mux  Inputs=6
  x,y,psi (Cars 1 - 6) : Outport
  wires:
  Demux/1 -> Extract x,y,psi/1(s,n,psi,us)
  Extract x,y,psi/1(x,y,psi) -> Mux/1
  Demux/2 -> Extract x,y,psi1/1(s,n,psi,us)
  Extract x,y,psi1/1(x,y,psi) -> Mux/2
  Demux/3 -> Extract x,y,psi2/1(s,n,psi,us)
  Extract x,y,psi2/1(x,y,psi) -> Mux/3
  Demux/4 -> Extract x,y,psi3/1(s,n,psi,us)
  Extract x,y,psi3/1(x,y,psi) -> Mux/4
  Demux/5 -> Extract x,y,psi4/1(s,n,psi,us)
  Extract x,y,psi4/1(x,y,psi) -> Mux/5
  s,n,psi,us (Cars 1 - 6)/1 -> Demux/1
  Mux/1 -> x,y,psi (Cars 1 - 6)/1
  Extract x,y,psi5/1(x,y,psi) -> Mux/6
  Demux/6 -> Extract x,y,psi5/1(s,n,psi,us)

== system Final_project_TEMPLATE/High Level Design/Outputs/Output Torque ==
  Torque : Inport
  Constant : Constant  Value=2e4
  Constant1 : Constant  Value=0.24
  Data Type Conversion : DataTypeConversion  OutDataTypeStr=uint32
  Data Type Conversion1 : DataTypeConversion  OutDataTypeStr=uint32
  Gain : Gain  Gain=100/0.52
  Saturation : Saturate  UpperLimit=822  LowerLimit=-822
  Simple PWM Output : rappid_564xl_ec_toolbox/MPC564xL/Motor Control Blocks/Simple PWM Output  Priority=1  pwmModule=0  pwmMod=0  SubModule=0  subMod=0  InitFreq=2e4  resolution=1 %  resValue=1  InitDutyA=50  InitDutyB=50  align=A B - center aligned  PhaseShift_A=0  PhaseShift=0  Phase_A=0  Phase_B=0  centered=1  DoubleS=off  doubleSw=off  debugSw=off  debug_mode=0  pin_A0=None  pin_B0="59  : PD11 : [ 78 ] : [ R16 ]"  pin_X0=None  pin_A1=None  pin_B1=None  pin_X1=None  pin_A2=None  pin_B2=None  pin_X2=None  pin_A3=None  pin_B3=None  pin_X3=None  pin1_A0=None  pin1_B0=None  pin1_X0=None  pin1_A1=None  pin1_B1=None  pin1_X1=None  pin1_A2=None  pin1_B2=None  pin1_X2=None  pin1_A3=None  pin1_B3=None  pin1_X3=None  pcrNumA=255  pcrNumB=59  pcrNumX=255  polA=off  polB=off  polX=off  octrl=0  syncFrom0=off  masterSync=0  outVal0=off  outVal1=off  outVal2=on  outVal3=on  outVal4=on  outVal5=on  outTrig=60
  Subsystem : Subsystem
  Sum : Sum  Inputs=|+-
  wires:
  Sum/1 -> Gain/1
  Gain/1 -> Data Type Conversion/1
  Data Type Conversion/1 -> Simple PWM Output/3, Simple PWM Output/2
  Data Type Conversion1/1 -> Simple PWM Output/1
  Constant/1 -> Data Type Conversion1/1
  Constant1/1 -> Sum/2
  Subsystem/1(Duty Cycle) -> Sum/1
  Torque/1 -> Saturation/1
  Saturation/1 -> Subsystem/1(Torque (Nmm))

== system Final_project_TEMPLATE/High Level Design/Outputs/Tx CAN ==
  s,n,psi,us : Inport
  CAN Transmit : rappid_564xl_ec_toolbox/MPC564xL/Communication Blocks/CAN Transmit  can_unit=A  can_unit_v2=0  can_buffer=15  can_id=35
  CAN Transmit1 : rappid_564xl_ec_toolbox/MPC564xL/Communication Blocks/CAN Transmit  can_unit=A  can_unit_v2=0  can_buffer=16  can_id=36
  Constant : Constant  Value=8  OutDataTypeStr=uint8
  Constant1 : Constant  Value=8  OutDataTypeStr=uint8
  Demux : Demux
  Mux : Mux  Inputs=2
  Mux1 : Mux  Inputs=2
  Single to Bytes{,1..3} (4 alike) : Conv_Lib/Single to Bytes
  wires:
  s,n,psi,us/1 -> Demux/1
  Demux/1 -> Single to Bytes/1
  Demux/2 -> Single to Bytes1/1
  Demux/3 -> Single to Bytes2/1
  Demux/4 -> Single to Bytes3/1
  Single to Bytes1/1 -> Mux/2
  Single to Bytes/1 -> Mux/1
  Mux1/1 -> CAN Transmit1/1
  Mux/1 -> CAN Transmit/1
  Constant1/1 -> CAN Transmit1/2
  Constant/1 -> CAN Transmit/2
  Single to Bytes2/1 -> Mux1/2
  Single to Bytes3/1 -> Mux1/1

== system Final_project_TEMPLATE/High Level Design/ACC/Speed Ctrl/PI ==
  Error : Inport
  Gain : Gain  Gain=V_Ki  SaturateOnIntegerOverflow=on  OutDataTypeStr=Inherit: Same as input  ParamDataTypeStr=Inherit: Same as input
  Gain1 : Gain  Gain=V_Kp  SaturateOnIntegerOverflow=on  OutDataTypeStr=Inherit: Same as input  ParamDataTypeStr=Inherit: Same as input
  My Discrete Integrator : Subsystem
  Sum : Sum  Inputs=|++  SaturateOnIntegerOverflow=on
  U : Outport
  wires:
  Sum/1 -> U/1
  Error/1 -> Gain1/1, Gain/1
  Gain1/1 -> Sum/2
  My Discrete Integrator/1(X) -> Sum/1
  Gain/1 -> My Discrete Integrator/1(X_dot)

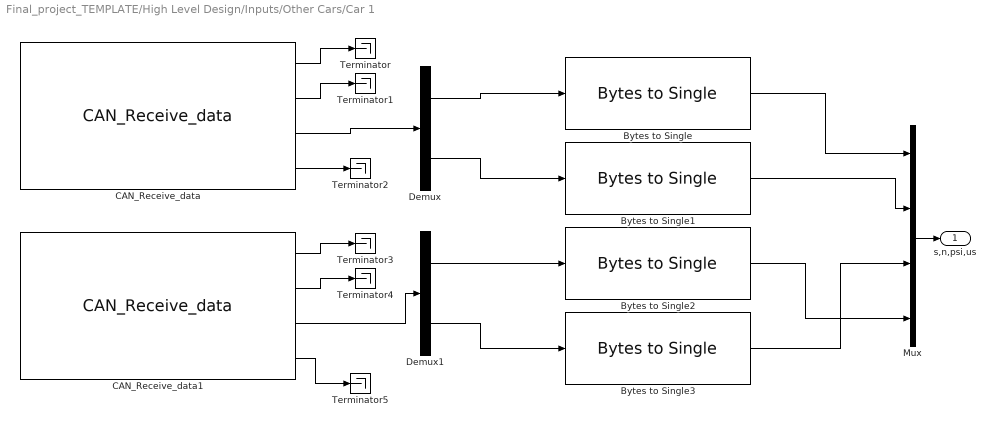
== system Final_project_TEMPLATE/High Level Design/Inputs/Other Cars/Car 1 ==
  Bytes to Single{,1..3} (4 alike) : Conv_Lib/Bytes to Single
  CAN_Receive_data : rappid_564xl_ec_toolbox/MPC564xL/Communication Blocks/CAN_Receive_data  can_unit=A  can_unit_v2=0  can_buffer=3  can_id=45
  CAN_Receive_data1 : rappid_564xl_ec_toolbox/MPC564xL/Communication Blocks/CAN_Receive_data  can_unit=A  can_unit_v2=0  can_buffer=4  can_id=46
  Demux : Demux  Outputs=2
  Demux1 : Demux  Outputs=2
  Mux : Mux
  Terminator{,1..5} (6 alike) : Terminator
  s,n,psi,us : Outport
  wires:
  Bytes to Single1/1 -> Mux/2
  Bytes to Single3/1 -> Mux/3
  Demux/1 -> Bytes to Single/1
  Demux/2 -> Bytes to Single1/1
  Demux1/1 -> Bytes to Single2/1
  Demux1/2 -> Bytes to Single3/1
  Bytes to Single/1 -> Mux/1
  Bytes to Single2/1 -> Mux/4
  Mux/1 -> s,n,psi,us/1
  CAN_Receive_data/1 -> Terminator/1
  CAN_Receive_data/2 -> Terminator1/1
  CAN_Receive_data/3 -> Demux/1
  CAN_Receive_data/4 -> Terminator2/1
  CAN_Receive_data1/1 -> Terminator3/1
  CAN_Receive_data1/2 -> Terminator4/1
  CAN_Receive_data1/3 -> Demux1/1
  CAN_Receive_data1/4 -> Terminator5/1

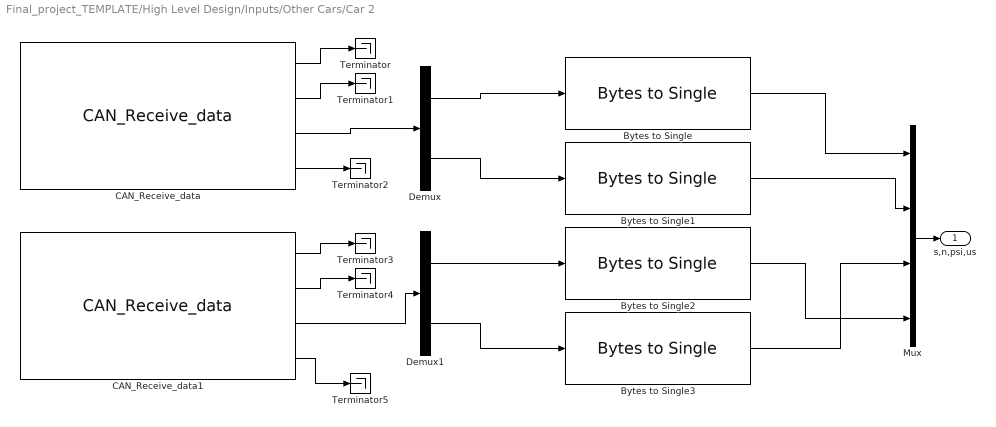
== system Final_project_TEMPLATE/High Level Design/Inputs/Other Cars/Car 2 ==
  Bytes to Single{,1..3} (4 alike) : Conv_Lib/Bytes to Single
  CAN_Receive_data : rappid_564xl_ec_toolbox/MPC564xL/Communication Blocks/CAN_Receive_data  can_unit=A  can_unit_v2=0  can_buffer=5  can_id=25
  CAN_Receive_data1 : rappid_564xl_ec_toolbox/MPC564xL/Communication Blocks/CAN_Receive_data  can_unit=A  can_unit_v2=0  can_buffer=6  can_id=26
  Demux : Demux  Outputs=2
  Demux1 : Demux  Outputs=2
  Mux : Mux
  Terminator{,1..5} (6 alike) : Terminator
  s,n,psi,us : Outport
  wires:
  Bytes to Single1/1 -> Mux/2
  Bytes to Single3/1 -> Mux/3
  Demux/1 -> Bytes to Single/1
  Demux/2 -> Bytes to Single1/1
  Demux1/1 -> Bytes to Single2/1
  Demux1/2 -> Bytes to Single3/1
  Bytes to Single/1 -> Mux/1
  Bytes to Single2/1 -> Mux/4
  Mux/1 -> s,n,psi,us/1
  CAN_Receive_data/1 -> Terminator/1
  CAN_Receive_data/2 -> Terminator1/1
  CAN_Receive_data/3 -> Demux/1
  CAN_Receive_data/4 -> Terminator2/1
  CAN_Receive_data1/1 -> Terminator3/1
  CAN_Receive_data1/2 -> Terminator4/1
  CAN_Receive_data1/3 -> Demux1/1
  CAN_Receive_data1/4 -> Terminator5/1

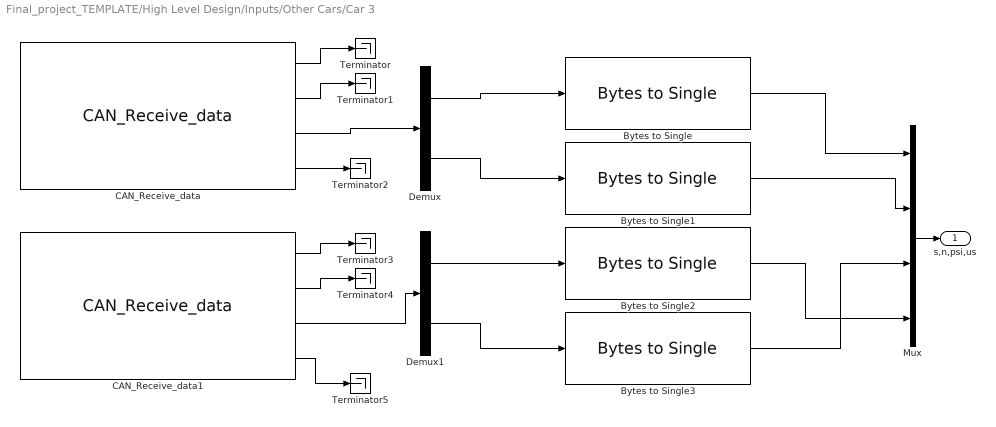
== system Final_project_TEMPLATE/High Level Design/Inputs/Other Cars/Car 3 ==
  Bytes to Single{,1..3} (4 alike) : Conv_Lib/Bytes to Single
  CAN_Receive_data : rappid_564xl_ec_toolbox/MPC564xL/Communication Blocks/CAN_Receive_data  can_unit=A  can_unit_v2=0  can_buffer=7  can_id=15
  CAN_Receive_data1 : rappid_564xl_ec_toolbox/MPC564xL/Communication Blocks/CAN_Receive_data  can_unit=A  can_unit_v2=0  can_buffer=8  can_id=16
  Demux : Demux  Outputs=2
  Demux1 : Demux  Outputs=2
  Mux : Mux
  Terminator{,1..5} (6 alike) : Terminator
  s,n,psi,us : Outport
  wires:
  Bytes to Single1/1 -> Mux/2
  Bytes to Single3/1 -> Mux/3
  Demux/1 -> Bytes to Single/1
  Demux/2 -> Bytes to Single1/1
  Demux1/1 -> Bytes to Single2/1
  Demux1/2 -> Bytes to Single3/1
  Bytes to Single/1 -> Mux/1
  Bytes to Single2/1 -> Mux/4
  Mux/1 -> s,n,psi,us/1
  CAN_Receive_data/1 -> Terminator/1
  CAN_Receive_data/2 -> Terminator1/1
  CAN_Receive_data/3 -> Demux/1
  CAN_Receive_data/4 -> Terminator2/1
  CAN_Receive_data1/1 -> Terminator3/1
  CAN_Receive_data1/2 -> Terminator4/1
  CAN_Receive_data1/3 -> Demux1/1
  CAN_Receive_data1/4 -> Terminator5/1

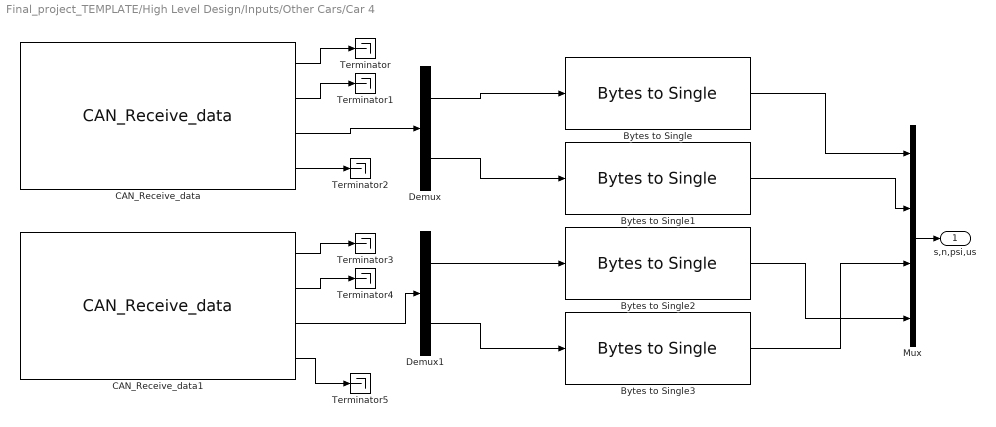
== system Final_project_TEMPLATE/High Level Design/Inputs/Other Cars/Car 4 ==
  Bytes to Single{,1..3} (4 alike) : Conv_Lib/Bytes to Single
  CAN_Receive_data : rappid_564xl_ec_toolbox/MPC564xL/Communication Blocks/CAN_Receive_data  can_unit=A  can_unit_v2=0  can_buffer=9  can_id=75
  CAN_Receive_data1 : rappid_564xl_ec_toolbox/MPC564xL/Communication Blocks/CAN_Receive_data  can_unit=A  can_unit_v2=0  can_buffer=10  can_id=76
  Demux : Demux  Outputs=2
  Demux1 : Demux  Outputs=2
  Mux : Mux
  Terminator{,1..5} (6 alike) : Terminator
  s,n,psi,us : Outport
  wires:
  Bytes to Single1/1 -> Mux/2
  Bytes to Single3/1 -> Mux/3
  Demux/1 -> Bytes to Single/1
  Demux/2 -> Bytes to Single1/1
  Demux1/1 -> Bytes to Single2/1
  Demux1/2 -> Bytes to Single3/1
  Bytes to Single/1 -> Mux/1
  Bytes to Single2/1 -> Mux/4
  Mux/1 -> s,n,psi,us/1
  CAN_Receive_data/1 -> Terminator/1
  CAN_Receive_data/2 -> Terminator1/1
  CAN_Receive_data/3 -> Demux/1
  CAN_Receive_data/4 -> Terminator2/1
  CAN_Receive_data1/1 -> Terminator3/1
  CAN_Receive_data1/2 -> Terminator4/1
  CAN_Receive_data1/3 -> Demux1/1
  CAN_Receive_data1/4 -> Terminator5/1

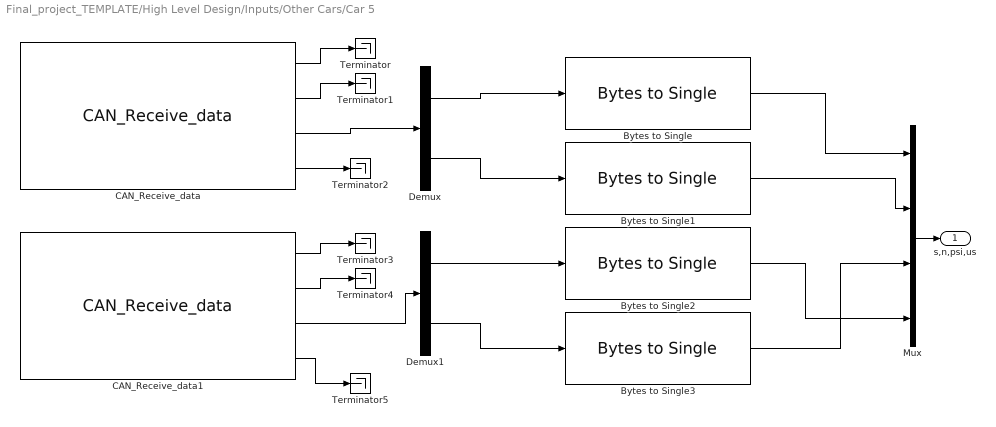
== system Final_project_TEMPLATE/High Level Design/Inputs/Other Cars/Car 5 ==
  Bytes to Single{,1..3} (4 alike) : Conv_Lib/Bytes to Single
  CAN_Receive_data : rappid_564xl_ec_toolbox/MPC564xL/Communication Blocks/CAN_Receive_data  can_unit=A  can_unit_v2=0  can_buffer=11  can_id=65
  CAN_Receive_data1 : rappid_564xl_ec_toolbox/MPC564xL/Communication Blocks/CAN_Receive_data  can_unit=A  can_unit_v2=0  can_buffer=12  can_id=66
  Demux : Demux  Outputs=2
  Demux1 : Demux  Outputs=2
  Mux : Mux
  Terminator{,1..5} (6 alike) : Terminator
  s,n,psi,us : Outport
  wires:
  Bytes to Single1/1 -> Mux/2
  Bytes to Single3/1 -> Mux/3
  Demux/1 -> Bytes to Single/1
  Demux/2 -> Bytes to Single1/1
  Demux1/1 -> Bytes to Single2/1
  Demux1/2 -> Bytes to Single3/1
  Bytes to Single/1 -> Mux/1
  Bytes to Single2/1 -> Mux/4
  Mux/1 -> s,n,psi,us/1
  CAN_Receive_data/1 -> Terminator/1
  CAN_Receive_data/2 -> Terminator1/1
  CAN_Receive_data/3 -> Demux/1
  CAN_Receive_data/4 -> Terminator2/1
  CAN_Receive_data1/1 -> Terminator3/1
  CAN_Receive_data1/2 -> Terminator4/1
  CAN_Receive_data1/3 -> Demux1/1
  CAN_Receive_data1/4 -> Terminator5/1

== system Final_project_TEMPLATE/High Level Design/Inputs/Other Cars/Car 6 ==
  Bytes to Single{,1..3} (4 alike) : Conv_Lib/Bytes to Single
  CAN_Receive_data : rappid_564xl_ec_toolbox/MPC564xL/Communication Blocks/CAN_Receive_data  can_unit=A  can_unit_v2=0  can_buffer=13  can_id=55
  CAN_Receive_data1 : rappid_564xl_ec_toolbox/MPC564xL/Communication Blocks/CAN_Receive_data  can_unit=A  can_unit_v2=0  can_buffer=14  can_id=56
  Demux : Demux  Outputs=2
  Demux1 : Demux  Outputs=2
  Mux : Mux
  Terminator{,1..5} (6 alike) : Terminator
  s,n,psi,us : Outport
  wires:
  Bytes to Single1/1 -> Mux/2
  Bytes to Single3/1 -> Mux/3
  Demux/1 -> Bytes to Single/1
  Demux/2 -> Bytes to Single1/1
  Demux1/1 -> Bytes to Single2/1
  Demux1/2 -> Bytes to Single3/1
  Bytes to Single/1 -> Mux/1
  Bytes to Single2/1 -> Mux/4
  Mux/1 -> s,n,psi,us/1
  CAN_Receive_data/1 -> Terminator/1
  CAN_Receive_data/2 -> Terminator1/1
  CAN_Receive_data/3 -> Demux/1
  CAN_Receive_data/4 -> Terminator2/1
  CAN_Receive_data1/1 -> Terminator3/1
  CAN_Receive_data1/2 -> Terminator4/1
  CAN_Receive_data1/3 -> Demux1/1
  CAN_Receive_data1/4 -> Terminator5/1

== system Final_project_TEMPLATE/High Level Design/Inputs/Other Cars/GSI Car (4)1 ==
  Bytes to Single{,1..3} (4 alike) : Conv_Lib/Bytes to Single
  CAN_Receive_data : rappid_564xl_ec_toolbox/MPC564xL/Communication Blocks/CAN_Receive_data  can_unit=A  can_unit_v2=0  can_buffer=0  can_id=105
  CAN_Receive_data1 : rappid_564xl_ec_toolbox/MPC564xL/Communication Blocks/CAN_Receive_data  can_unit=A  can_unit_v2=0  can_buffer=1  can_id=106
  Demux : Demux  Outputs=2
  Demux1 : Demux  Outputs=2
  Mux : Mux
  Terminator{,1..5} (6 alike) : Terminator
  s,n,psi,us : Outport
  wires:
  Bytes to Single1/1 -> Mux/2
  Bytes to Single3/1 -> Mux/3
  Demux/1 -> Bytes to Single/1
  Demux/2 -> Bytes to Single1/1
  Demux1/1 -> Bytes to Single2/1
  Demux1/2 -> Bytes to Single3/1
  Bytes to Single/1 -> Mux/1
  Bytes to Single2/1 -> Mux/4
  Mux/1 -> s,n,psi,us/1
  CAN_Receive_data/1 -> Terminator/1
  CAN_Receive_data/2 -> Terminator1/1
  CAN_Receive_data/3 -> Demux/1
  CAN_Receive_data/4 -> Terminator2/1
  CAN_Receive_data1/1 -> Terminator3/1
  CAN_Receive_data1/2 -> Terminator4/1
  CAN_Receive_data1/3 -> Demux1/1
  CAN_Receive_data1/4 -> Terminator5/1

== system Final_project_TEMPLATE/High Level Design/Inputs/Other Cars/Zeros (20)1 ==
  Constant : Constant  Value=0  OutDataTypeStr=single
  Mux : Mux  Inputs=20
  Zeros : Outport
  wires:
  Mux/1 -> Zeros/1
  Constant/1 -> Mux/1, Mux/2, Mux/3, Mux/4, Mux/5, Mux/6, Mux/7, Mux/8, Mux/9, Mux/10, Mux/11, Mux/13, Mux/16, Mux/17, Mux/18, Mux/19, Mux/20, Mux/15, Mux/14, Mux/12

== system Final_project_TEMPLATE/High Level Design/Inputs/Steering angle (QD)/Conversion Subsystem ==
  Encoder Counts : Inport
  Data Type Conversion : DataTypeConversion  OutDataTypeStr=uint16
  Data Type Conversion1 : DataTypeConversion  OutDataTypeStr=int16
  Data Type Conversion2 : DataTypeConversion  OutDataTypeStr=single
  Delay : Delay  DelayLength=1  InitialCondition=0
  Delay1 : Delay  DelayLength=1  InitialCondition=0
  Gain : Gain  Gain=t2d
  Sum : Sum  Inputs=|+-
  Sum1 : Sum  Inputs=|++
  Haptic Wheel Position (degree) : Outport
  wires:
  Data Type Conversion/1 -> Delay/1, Sum/1
  Encoder Counts/1 -> Data Type Conversion/1
  Sum/1 -> Data Type Conversion1/1
  Delay/1 -> Sum/2
  Gain/1 -> Sum1/1
  Data Type Conversion2/1 -> Gain/1
  Delay1/1 -> Sum1/2
  Data Type Conversion1/1 -> Data Type Conversion2/1
  Sum1/1 -> Haptic Wheel Position (degree)/1, Delay1/1

== system Final_project_TEMPLATE/High Level Design/Outputs/Extract x,y,psi (Cars 1 - 6)/Extract x,y,psi ==
  s,n,psi,us : Inport
  Demux : Demux
  Mux : Mux  Inputs=3
  Terminator : Terminator
  s,n to x,y : Veh_Sim/s,n to x,y  SystemSampleTime=-1
  x,y,psi : Outport
  wires:
  Demux/1 -> s,n to x,y/1
  Demux/2 -> s,n to x,y/2
  s,n,psi,us/1 -> Demux/1
  s,n to x,y/1 -> Mux/1
  s,n to x,y/2 -> Mux/2
  Demux/3 -> Mux/3
  Mux/1 -> x,y,psi/1
  Demux/4 -> Terminator/1

== system Final_project_TEMPLATE/High Level Design/Outputs/Extract x,y,psi (Cars 1 - 6)/Extract x,y,psi1 ==
  s,n,psi,us : Inport
  Demux : Demux
  Mux : Mux  Inputs=3
  Terminator : Terminator
  s,n to x,y : Veh_Sim/s,n to x,y  SystemSampleTime=-1
  x,y,psi : Outport
  wires:
  Demux/1 -> s,n to x,y/1
  Demux/2 -> s,n to x,y/2
  s,n,psi,us/1 -> Demux/1
  s,n to x,y/1 -> Mux/1
  s,n to x,y/2 -> Mux/2
  Demux/3 -> Mux/3
  Mux/1 -> x,y,psi/1
  Demux/4 -> Terminator/1

== system Final_project_TEMPLATE/High Level Design/Outputs/Extract x,y,psi (Cars 1 - 6)/Extract x,y,psi2 ==
  s,n,psi,us : Inport
  Demux : Demux
  Mux : Mux  Inputs=3
  Terminator : Terminator
  s,n to x,y : Veh_Sim/s,n to x,y  SystemSampleTime=-1
  x,y,psi : Outport
  wires:
  Demux/1 -> s,n to x,y/1
  Demux/2 -> s,n to x,y/2
  s,n,psi,us/1 -> Demux/1
  s,n to x,y/1 -> Mux/1
  s,n to x,y/2 -> Mux/2
  Demux/3 -> Mux/3
  Mux/1 -> x,y,psi/1
  Demux/4 -> Terminator/1

== system Final_project_TEMPLATE/High Level Design/Outputs/Extract x,y,psi (Cars 1 - 6)/Extract x,y,psi3 ==
  s,n,psi,us : Inport
  Demux : Demux
  Mux : Mux  Inputs=3
  Terminator : Terminator
  s,n to x,y : Veh_Sim/s,n to x,y  SystemSampleTime=-1
  x,y,psi : Outport
  wires:
  Demux/1 -> s,n to x,y/1
  Demux/2 -> s,n to x,y/2
  s,n,psi,us/1 -> Demux/1
  s,n to x,y/1 -> Mux/1
  s,n to x,y/2 -> Mux/2
  Demux/3 -> Mux/3
  Mux/1 -> x,y,psi/1
  Demux/4 -> Terminator/1

== system Final_project_TEMPLATE/High Level Design/Outputs/Extract x,y,psi (Cars 1 - 6)/Extract x,y,psi4 ==
  s,n,psi,us : Inport
  Demux : Demux
  Mux : Mux  Inputs=3
  Terminator : Terminator
  s,n to x,y : Veh_Sim/s,n to x,y  SystemSampleTime=-1
  x,y,psi : Outport
  wires:
  Demux/1 -> s,n to x,y/1
  Demux/2 -> s,n to x,y/2
  s,n,psi,us/1 -> Demux/1
  s,n to x,y/1 -> Mux/1
  s,n to x,y/2 -> Mux/2
  Demux/3 -> Mux/3
  Mux/1 -> x,y,psi/1
  Demux/4 -> Terminator/1

== system Final_project_TEMPLATE/High Level Design/Outputs/Extract x,y,psi (Cars 1 - 6)/Extract x,y,psi5 ==
  s,n,psi,us : Inport
  Demux : Demux
  Mux : Mux  Inputs=3
  Terminator : Terminator
  s,n to x,y : Veh_Sim/s,n to x,y  SystemSampleTime=-1
  x,y,psi : Outport
  wires:
  Demux/1 -> s,n to x,y/1
  Demux/2 -> s,n to x,y/2
  s,n,psi,us/1 -> Demux/1
  s,n to x,y/1 -> Mux/1
  s,n to x,y/2 -> Mux/2
  Demux/3 -> Mux/3
  Mux/1 -> x,y,psi/1
  Demux/4 -> Terminator/1

== system Final_project_TEMPLATE/High Level Design/Outputs/Output Torque/Subsystem ==
  Torque (Nmm) : Inport
  Add : Sum
  Constant : Constant  Value=0.5
  Gain : Gain  Gain=3.162e-4
  Saturation : Saturate  UpperLimit=dc_sathigh  LowerLimit=dc_satlow
  Duty Cycle : Outport
  wires:
  Gain/1 -> Add/2
  Torque (Nmm)/1 -> Gain/1
  Constant/1 -> Add/1
  Add/1 -> Saturation/1
  Saturation/1 -> Duty Cycle/1
